simulink library "INT_OilP_DD"  (R2016b)
settings: Solver=VariableStepAuto  StartTime=0.0  StopTime=10.0  RelTol=1e-3
settings Model: Creator=xinchangran  LastModifiedBy=xinchangran

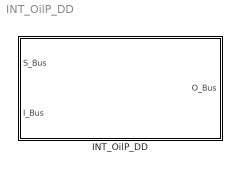
== system INT_OilP_DD ==
  INT_OilP_DD : Subsystem

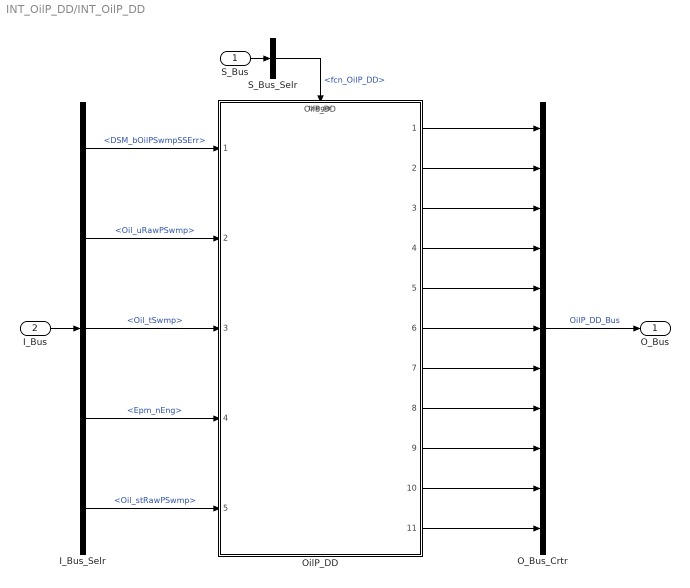
== system INT_OilP_DD/INT_OilP_DD ==
  S_Bus : Inport
  I_Bus : Inport  Port=2
  I_Bus_Selr : BusSelector  OutputSignals=DSM_bOilPSwmpSSErr,Oil_uRawPSwmp,Oil_tSwmp,Epm_nEng,Oil_stRawPSwmp
  O_Bus_Crtr : BusCreator  Inputs=11
  OilP_DD : ModelReference  ModelNameDialog=OilP_DD  SimulationMode=Normal  ModelReferenceVersion=1.41  TriggerPortName=function  TriggerPortTriggerType=function-call  TriggerPortStatesWhenEnabling=held
  S_Bus_Selr : BusSelector  OutputSignals=fcn_OilP_DD
  O_Bus : Outport
  wires:
  S_Bus_Selr/1 -> OilP_DD/Trigger  "<fcn_OilP_DD>"
  S_Bus/1 -> S_Bus_Selr/1
  I_Bus/1 -> I_Bus_Selr/1
  I_Bus_Selr/1 -> OilP_DD/1  "<DSM_bOilPSwmpSSErr>"
  I_Bus_Selr/2 -> OilP_DD/2  "<Oil_uRawPSwmp>"
  I_Bus_Selr/3 -> OilP_DD/3  "<Oil_tSwmp>"
  I_Bus_Selr/4 -> OilP_DD/4  "<Epm_nEng>"
  I_Bus_Selr/5 -> OilP_DD/5  "<Oil_stRawPSwmp>"
  O_Bus_Crtr/1 -> O_Bus/1  "OilP_DD_Bus"
  OilP_DD/1 -> O_Bus_Crtr/1
  OilP_DD/2 -> O_Bus_Crtr/2
  OilP_DD/3 -> O_Bus_Crtr/3
  OilP_DD/4 -> O_Bus_Crtr/4
  OilP_DD/5 -> O_Bus_Crtr/5
  OilP_DD/6 -> O_Bus_Crtr/6
  OilP_DD/7 -> O_Bus_Crtr/7
  OilP_DD/8 -> O_Bus_Crtr/8
  OilP_DD/9 -> O_Bus_Crtr/9
  OilP_DD/10 -> O_Bus_Crtr/10
  OilP_DD/11 -> O_Bus_Crtr/11
